simulink model "OpenDiscon_block"  (Simulink 8.3)
settings: Solver=ode45  StartTime=0.0  StopTime=10.0  RelTol=1e-3
settings Model: Creator=ielorza  LastModifiedBy=ielorza
settings DataIOCC: SignalLoggingSaveFormat=Dataset
settings DebuggingCC: UnderspecifiedInitializationDetection=Simplified  StateNameClashWarn=none
settings GRTTargetCC: CombineOutputUpdateFcns=on  GRTInterface=off

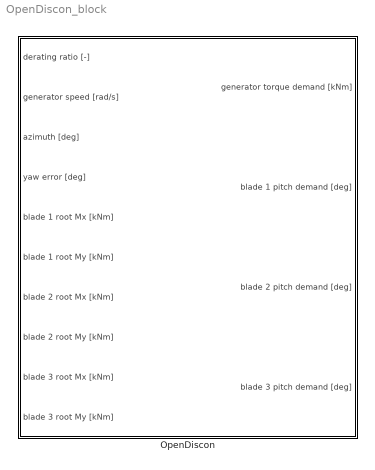
== system OpenDiscon_block ==
  OpenDiscon : Subsystem

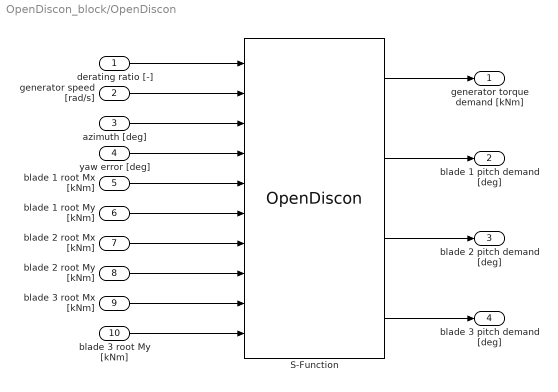
== system OpenDiscon_block/OpenDiscon ==
  derating ratio [-] : Inport
  generator speed [rad/s] : Inport  Port=2
  azimuth [deg] : Inport  Port=3
  yaw error [deg] : Inport  Port=4
  blade 1 root Mx [kNm] : Inport  Port=5
  blade 1 root My [kNm] : Inport  Port=6
  blade 2 root Mx [kNm] : Inport  Port=7
  blade 2 root My [kNm] : Inport  Port=8
  blade 3 root Mx [kNm] : Inport  Port=9
  blade 3 root My [kNm] : Inport  Port=10
  S-Function : S-Function  FunctionName=OpenDiscon  EnableBusSupport=off
  generator torque demand [kNm] : Outport
  blade 1 pitch demand [deg] : Outport  Port=2
  blade 2 pitch demand [deg] : Outport  Port=3
  blade 3 pitch demand [deg] : Outport  Port=4
  wires:
  derating ratio [-]/1 -> S-Function/1
  azimuth [deg]/1 -> S-Function/3
  blade 2 root My [kNm]/1 -> S-Function/8
  blade 3 root Mx [kNm]/1 -> S-Function/9
  yaw error [deg]/1 -> S-Function/4
  blade 1 root Mx [kNm]/1 -> S-Function/5
  blade 1 root My [kNm]/1 -> S-Function/6
  blade 2 root Mx [kNm]/1 -> S-Function/7
  generator speed [rad/s]/1 -> S-Function/2
  blade 3 root My [kNm]/1 -> S-Function/10
  S-Function/4 -> blade 3 pitch demand [deg]/1
  S-Function/3 -> blade 2 pitch demand [deg]/1
  S-Function/2 -> blade 1 pitch demand [deg]/1
  S-Function/1 -> generator torque demand [kNm]/1
